simulink model "ppfir5"  (R2012b)
(part 2 of 79)

  Delay144/1 -> mixer3/2(dds_in)
  Delay147/1 -> Logical/2
  Delay148/1 -> Logical/1
  Delay151/1 -> Delay16/1
  Slice7/1 -> pipeline1/1(d)
  pipeline1/1(q) -> Relational5/1
  pipeline2/1(q) -> Delay60/1
  Slice3/1 -> pipeline2/1(d)
  pipeline3/1(q) -> Relational6/2
  pipeline4/1(q) -> Mux1/1, Mux2/1
  pipeline5/1(q) -> dds_delay/2(delay)
  pipeline6/1(q) -> dds_delay/1(din)
  pipeline23/1(q) -> bus_expand1/1(bus_in)
  Mux3/1 -> Terminator1/1
  Relational/1 -> Terminator4/1
  Mux2/1 -> Terminator5/1
  Mux1/1 -> Terminator8/1
  pipeline8/1(q) -> Delay47/1, Delay38/1, edge_detect/1(in)
  pipeline9/1(q) -> photonDataOut0/1(out_reg)
  pipeline10/1(q) -> we_out0/1(out_reg)
  pipeline11/1(q) -> photonDataOut1/1(out_reg)
  pipeline12/1(q) -> we_out1/1(out_reg)
  pipeline13/1(q) -> photonDataOut2/1(out_reg)
  pipeline14/1(q) -> we_out2/1(out_reg)
  pipeline15/1(q) -> photonDataOut3/1(out_reg)
  pipeline16/1(q) -> we_out3/1(out_reg)
  pipeline17/1(q) -> avgIQ/2(trig), avgIQ1/2(trig), avgIQ3/2(trig), avgIQ2/2(trig), posedge/1(in)
  pipeline18/1(q) -> pfb_fft/1(data_in)
  Delay11/1 -> pfb_fft/2(sync_in)
  Delay14/1 -> Delay45/1, chan_sel/1(bin_ctr)
  pipeline21/1(q) -> Delay39/1, chan_sel/2(fft_data)
  Delay12/1 -> chan_sel/3(fft_rdy)
